simulink model "SteeringColumn"  (R2023a)
settings: Solver=VariableStepAuto  StartTime=0.0  StopTime=10.0  RelTol=1e-3
undefined symbols (not defined in the file): c, C1, C2, J1, J2, K, T_f
settings Model: Creator=Tan_Tram  LastModifiedBy=Tan_Tram

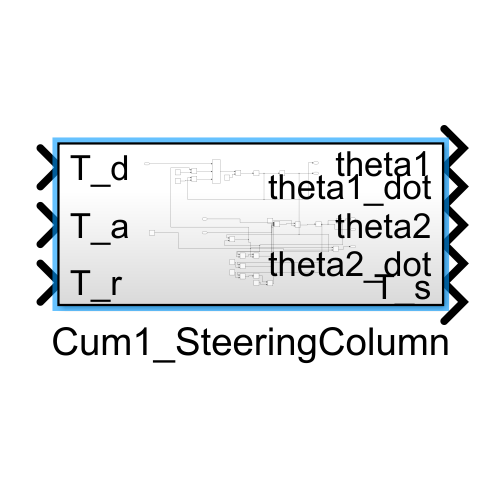
[thumbnail: Simulink's stored preview of the top-level diagram]
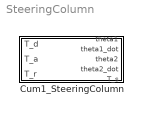
== system SteeringColumn ==
  Cum1_SteeringColumn : Subsystem

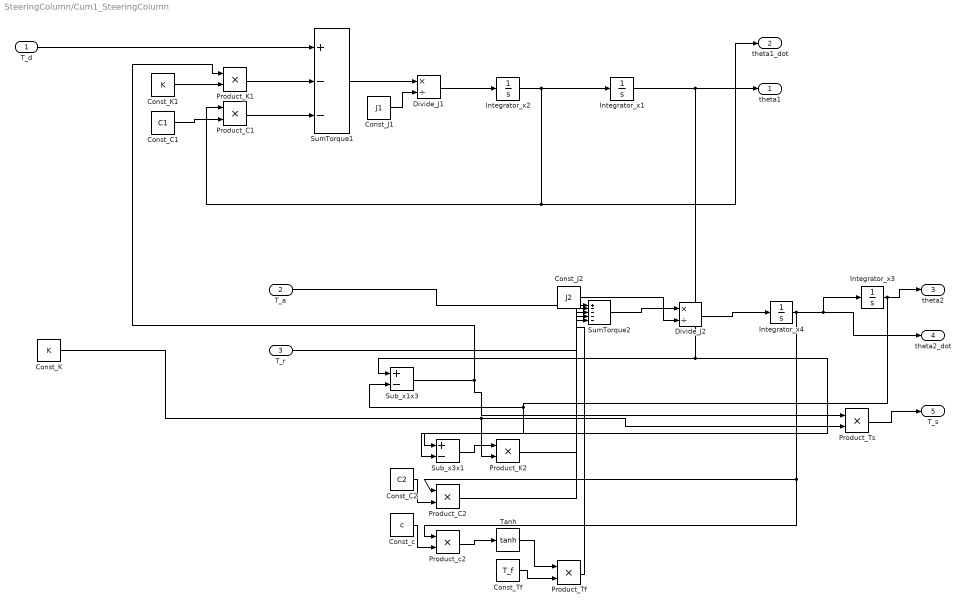
== system SteeringColumn/Cum1_SteeringColumn ==
  T_d : Inport
  T_a : Inport  Port=2
  T_r : Inport  Port=3
  Const_C1 : Constant  Value=C1
  Const_C2 : Constant  Value=C2
  Const_J1 : Constant  Value=J1
  Const_J2 : Constant  Value=J2
  Const_K : Constant  Value=K
  Const_K1 : Constant  Value=K
  Const_Tf : Constant  Value=T_f
  Const_c : Constant  Value=c
  Divide_J1 : Product  Inputs=*/
  Divide_J2 : Product  Inputs=*/
  Integrator_x{1..4} (4 alike) : Integrator
  Product_C1 : Product
  Product_C2 : Product
  Product_K1 : Product
  Product_K2 : Product
  Product_Tf : Product
  Product_Ts : Product
  Product_c2 : Product
  Sub_x1x3 : Sum  Inputs=+-
  Sub_x3x1 : Sum  Inputs=+-
  SumTorque1 : Sum  Inputs=+--
  SumTorque2 : Sum  Inputs=+----
  Tanh : Trigonometry  Operator=tanh
  theta1 : Outport
  theta1_dot : Outport  Port=2
  theta2 : Outport  Port=3
  theta2_dot : Outport  Port=4
  T_s : Outport  Port=5
  wires:
  Integrator_x1/1 -> theta1/1, Sub_x3x1/2, Sub_x1x3/1
  Integrator_x3/1 -> Sub_x1x3/2, Sub_x3x1/1, theta2/1
  Sub_x1x3/1 -> Product_K1/1, Product_Ts/1
  Const_K/1 -> Product_Ts/2, Product_K2/2
  Integrator_x2/1 -> theta1_dot/1, Product_C1/1, Integrator_x1/1
  Const_C1/1 -> Product_C1/2
  T_d/1 -> SumTorque1/1
  Product_K1/1 -> SumTorque1/2
  Product_C1/1 -> SumTorque1/3
  SumTorque1/1 -> Divide_J1/1
  Const_J1/1 -> Divide_J1/2
  Divide_J1/1 -> Integrator_x2/1
  Sub_x3x1/1 -> Product_K2/1
  Integrator_x4/1 -> Product_C2/1, Product_c2/1, Integrator_x3/1, theta2_dot/1
  Const_C2/1 -> Product_C2/2
  Const_c/1 -> Product_c2/2
  Product_c2/1 -> Tanh/1
  Tanh/1 -> Product_Tf/1
  Const_Tf/1 -> Product_Tf/2
  T_a/1 -> SumTorque2/1
  T_r/1 -> SumTorque2/2
  Product_Tf/1 -> SumTorque2/3
  Product_C2/1 -> SumTorque2/4
  Product_K2/1 -> SumTorque2/5
  SumTorque2/1 -> Divide_J2/1
  Const_J2/1 -> Divide_J2/2
  Divide_J2/1 -> Integrator_x4/1
  Product_Ts/1 -> T_s/1
  Const_K1/1 -> Product_K1/2
